simulink model "OrientationAnimationModel"  (R2023b)
settings: Solver=ode3  StartTime=0.0  StopTime=500  FixedStep=.010  RelTol=1e-3
model workspace (MAT data in the model file):
  B = Simulink.Parameter
  B.Value = Simulink.data.Expression
  B.Value.ExpressionString = "3.42*(1e-6)/((2*pi/60)*1e3)"
  B.DataType = 'auto'
  B.Complexity = 'real'
  B.Dimensions = -1
  J = Simulink.Parameter
  J.Value = Simulink.data.Expression
  J.Value.ExpressionString = "0.5*0.05*(0.05)^2"
  J.DataType = 'auto'
  J.Complexity = 'real'
  J.Dimensions = -1
  Kt = Simulink.Parameter
  Kt.Value = Simulink.data.Expression
  Kt.Value.ExpressionString = "3.56*1e-3"
  Kt.DataType = 'auto'
  Kt.Complexity = 'real'
  Kt.Dimensions = -1
  L = Simulink.Parameter
  L.Value = Simulink.data.Expression
  L.Value.ExpressionString = "570*1e-6"
  L.DataType = 'auto'
  L.Complexity = 'real'
  L.Dimensions = -1
  M1_Gain = Simulink.Parameter
  M1_Gain.Value = 8.4
  M1_Gain.DataType = 'auto'
  M1_Gain.Complexity = 'real'
  M1_Gain.Dimensions = [1 1]
  M1_I_max = Simulink.Parameter
  M1_I_max.Value = 0.075
  M1_I_max.DataType = 'auto'
  M1_I_max.Complexity = 'real'
  M1_I_max.Dimensions = [1 1]
  M1_V = Simulink.Parameter
  M1_V.Value = 5
  M1_V.DataType = 'auto'
  M1_V.Complexity = 'real'
  M1_V.Dimensions = [1 1]
  M2_Gain = Simulink.Parameter
  M2_Gain.Value = 8.4
  M2_Gain.DataType = 'auto'
  M2_Gain.Complexity = 'real'
  M2_Gain.Dimensions = [1 1]
  M2_I_max = Simulink.Parameter
  M2_I_max.Value = 0.075
  M2_I_max.DataType = 'auto'
  M2_I_max.Complexity = 'real'
  M2_I_max.Dimensions = [1 1]
  M2_V = Simulink.Parameter
  M2_V.Value = 5
  M2_V.DataType = 'auto'
  M2_V.Complexity = 'real'
  M2_V.Dimensions = [1 1]
  R = Simulink.Parameter
  R.Value = Simulink.data.Expression
  R.Value.ExpressionString = "22"
  R.DataType = 'auto'
  R.Complexity = 'real'
  R.Dimensions = -1
  orbit_altitude = 450000
  r_earth = 6378100
  vel_init = 7640
undefined symbols (not defined in the file or in its folder): m1, m2, m3, V1, V2, V3
libraries: aerolibutil x5, dspinverses x4, sharedtransform x4, simulink x3, vrlib x1, dspmtrx3 x1, matrix_library x1, spsSampleandHoldLib x1
settings Model: SnapshotInterval=1  Creator=Ian Lee  LastModifiedBy=andrea
settings DebuggingCC: UnconnectedInputMsg=warning  UnconnectedOutputMsg=warning  UnconnectedLineMsg=warning
settings ModelReferenceCC: EnableRefExpFcnMdlSchedulingChecks=on  ModelReferenceMinAlgLoopOccurrences=on
settings RTWCC: DLArmComputeVersion=19.05

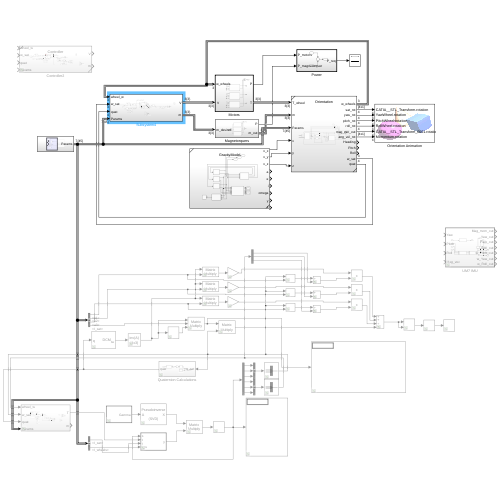
[thumbnail: Simulink's stored preview of the top-level diagram]
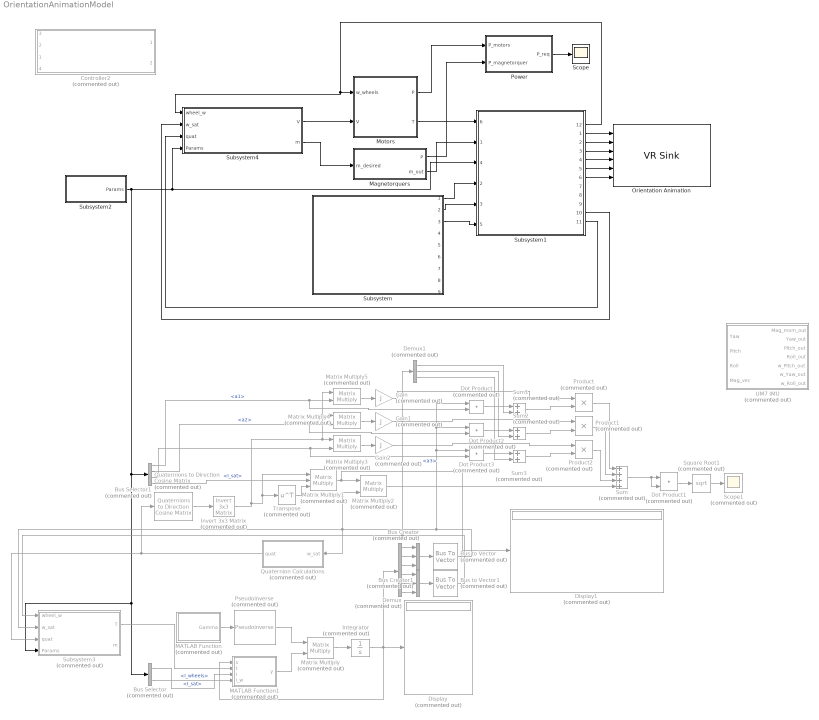
== system OrientationAnimationModel ==
  Bus Creator : BusCreator  Commented=on  Inputs=3
  Bus Creator1 : BusCreator  Commented=on  Inputs=3
  Bus Selector : BusSelector  Commented=on  OutputSignals=I_sat,I_wheels
  Bus Selector1 : BusSelector  Commented=on  OutputSignals=a1,a2,a3,I_sat
  Bus to Vector : BusToVector  Commented=on
  Bus to Vector1 : BusToVector  Commented=on
  Controller2 : Subsystem  Commented=on  ReferencedSubsystem=Controller
      settings: PortSchema="{\"entries\":[{\"content\":{\"sides\":[{\"content\":{\"connectorIds\":[\"In3\",\"In2\",\"In1\",\"In4\"]},\"type\":\"ConnectorPlacement.EquallySpacedRectSide\",\"uuid\":\"79f889b4-4a86-42cb-9f90-6ea385053cf3\"},{\"content\":{\"connectorIds\":[\"Out1\",\"Out2\"],\"side\":\"RIGHT\"},\"type\":\"ConnectorPlacement.EquallySpacedRectSide\",\"uuid\":\"c6c22cdf-cbb6-43f0-a5d1-c6e13417ad06\"},{\"content\":{\"side\":\"TOP\"},\"type\":\"ConnectorPlacement.EquallySpacedRectSide\",\"uuid\":\"fe3f8c93-2b15-4833-a3bc-63f563fd4268\"}]},\"type\":\"ConnectorPlacement.EquallySpacedConnector\",\"uuid\":\"198af49c-de07-4ebb-ae2e-d5790619fe38\"}],\"packageUris\":[\"http://schema.mathworks.com/mf0/Connector/R2020b\"],\"version\":\"1.0\"}"
  Demux : Demux  Commented=on  Outputs=6
  Demux1 : Demux  Commented=on  Outputs=3
  Display : Display  Commented=on
  Display1 : Display  Commented=on
  Dot Product{,1..3} (4 alike) : DotProduct  Commented=on  OutDataTypeStr=Inherit: Inherit via internal rule
  Gain : Gain  Commented=on  Gain=J
  Gain1 : Gain  Commented=on  Gain=J
  Gain2 : Gain  Commented=on  Gain=J
  Integrator : Integrator  Commented=on  InitialCondition=[0;0;0;0;0;0]
  Invert 3x3 Matrix : aerolibutil/Invert  3x3 Matrix  Commented=on
  MATLAB Function : MATLAB Function  Commented=on  TreatAsAtomicUnit=on
  MATLAB Function1 : MATLAB Function  Commented=on  TreatAsAtomicUnit=on
  Magnetorquers : Subsystem
  Matrix Multiply{,2..5} (5 alike) : Product  Commented=on  Multiplication=Matrix(*)
  Matrix Multiply1 : Product  Commented=on  Inputs=3  Multiplication=Matrix(*)
  Motors : Subsystem  TreatAsAtomicUnit=on
  Orientation Animation : vrlib/VR Sink  InstantiateOnLoad=on  SampleTime=.02  ViewEnable=on  RemoteChange=off  RemoteView=off  FieldsWritten=CATIA__STL_Transform.rotation.4.1.1.double#YawWheel.rotation.4.1.1.double#PitchWheel.rotation.4.1.1.double#RollWheel.rotation.4.1.1.double#CATIA__STL_Transform_0001.rotation.4.1.1.double#Momentum.rotation.4.1.1.double  WorldFileName=SatVR.x3d  AutoView=off  VideoDimensions=[]  AllowVariableSize=off
  Power : Subsystem  TreatAsAtomicUnit=on
  Product : Product  Commented=on
  Product1 : Product  Commented=on
  Product2 : Product  Commented=on
  Pseudoinverse : dspinverses/Pseudoinverse  Commented=on  wanterr=off  SimulateUsing=Interpreted execution
  Quaternion Calculations : Subsystem  Commented=on
  Quaternions to Direction Cosine Matrix : sharedtransform/Quaternions to  Direction Cosine Matrix  Commented=on  aMode=aMode
      settings: LibrarySourceBlock=|
      | aerolibtransform2/Quaternions to
      | Direction Cosine Matrix
  Scope : Scope
  Scope1 : Scope  Commented=on
  Square Root1 : Sqrt  Commented=on
  Subsystem : Subsystem  ReferencedSubsystem=GravityModel
  Subsystem1 : Subsystem  ReferencedSubsystem=Orientation
      settings: PortSchema="{\"entries\":[{\"content\":{\"sides\":[{\"content\":{\"connectorIds\":[\"In6\",\"In1\",\"In4\",\"In2\",\"In3\",\"In5\"]},\"type\":\"ConnectorPlacement.EquallySpacedRectSide\",\"uuid\":\"8242cc14-2b60-48ca-86c2-9381cf9d168d\"},{\"content\":{\"connectorIds\":[\"Out12\",\"Out1\",\"Out2\",\"Out3\",\"Out4\",\"Out5\",\"Out6\",\"Out7\",\"Out8\",\"Out9\",\"Out10\",\"Out11\"],\"side\":\"RIGHT\"},\"type\":\"ConnectorPlacement.EquallySpacedRectSide\",\"uuid\":\"8dac9f9e-c84b-46a7-8096-472338eb4c0b\"},{\"content\":{\"side\":\"TOP\"},\"type\":\"ConnectorPlacement.EquallySpacedRectSide\",\"uuid\":\"ad35a777-644b-4799-a01f-486ba56fdd07\"}]},\"type\":\"ConnectorPlacement.EquallySpacedConnector\",\"uuid\":\"a47ae8ba-a922-42d0-80de-66716a9fad33\"}],\"packageUris\":[\"http://schema.mathworks.com/mf0/Connector/R2020b\"],\"version\":\"1.0\"}"
  Subsystem2 : Subsystem
  Subsystem3 : Subsystem  Commented=on
  Subsystem4 : Subsystem
  Sum : Sum  Commented=on  Inputs=++++
  Sum1 : Sum  Commented=on
  Sum2 : Sum  Commented=on
  Sum3 : Sum  Commented=on
  Transpose : Math  Commented=on  Operator=transpose
  UM7 IMU : Subsystem  Commented=on  TreatAsAtomicUnit=on
  wires:
  Subsystem/1 -> Subsystem1/2
  Subsystem/2 -> Subsystem1/3
  Subsystem/3 -> Subsystem1/5
  Power/1(P_req) -> Scope/1
  Magnetorquers/1(P) -> Power/2(P_magnetorquer)
  Subsystem1/1 -> Orientation Animation/1
  Subsystem1/2 -> Orientation Animation/2
  Subsystem1/3 -> Orientation Animation/3
  Subsystem1/4 -> Orientation Animation/4
  Subsystem1/5 -> Orientation Animation/5
  Subsystem1/6 -> Orientation Animation/6
  Subsystem1/11 -> Subsystem4/3(quat)
  Subsystem1/10 -> Subsystem4/2(w_sat)
  Subsystem4/1(V) -> Motors/2(" V")
  Subsystem4/2(m) -> Magnetorquers/1(m_desired)
  Magnetorquers/2(m_out) -> Subsystem1/1
  Motors/1(P) -> Power/1(P_motors)
  Motors/2(T) -> Subsystem1/6
  Subsystem1/12 -> Subsystem4/1(wheel_w), Motors/1(w_wheels)
  Subsystem2/1(Params) -> Subsystem4/4(Params), Subsystem1/4, Bus Selector1/1, Subsystem3/4(Params), Bus Selector/1
  MATLAB Function/1(Gamma) -> Pseudoinverse/1
  Pseudoinverse/1 -> Matrix Multiply/1
  MATLAB Function1/1(y) -> Matrix Multiply/2
  Matrix Multiply/1 -> Integrator/1
  Integrator/1 -> Demux/1, MATLAB Function1/1(s), Display/1
  Bus Selector/1 -> MATLAB Function1/3(I)  "<I_sat>"
  Bus Selector/2 -> MATLAB Function1/4(I_w)  "<I_wheels>"
  Demux/1 -> Bus Creator/1
  Demux/2 -> Bus Creator/2
  Demux/3 -> Bus Creator/3
  Demux/4 -> Bus Creator1/1
  Demux/5 -> Bus Creator1/2
  Demux/6 -> Bus Creator1/3
  Bus Creator/1 -> Bus to Vector/1
  Bus Creator1/1 -> Bus to Vector1/1
  Bus to Vector/1 -> Dot Product3/1, Dot Product2/1, Dot Product/1, Matrix Multiply2/2, Quaternion Calculations/1(w_sat), Subsystem3/2(w_sat)
  Bus to Vector1/1 -> Demux1/1, Subsystem3/1(wheel_w)
  Quaternion Calculations/1(quat) -> Quaternions to Direction Cosine Matrix/1, Subsystem3/3(quat)
  Subsystem3/1(T) -> MATLAB Function1/2(t)
  Transpose/1 -> Matrix Multiply1/3
  Matrix Multiply1/1 -> Display1/1, Matrix Multiply2/1
  Bus Selector1/4 -> Matrix Multiply1/2  "<I_sat>"
  Bus Selector1/3 -> Dot Product3/2, Matrix Multiply3/2  "<a3>"
  Bus Selector1/2 -> Dot Product2/2, Matrix Multiply4/2  "<a2>"
  Bus Selector1/1 -> Dot Product/2, Matrix Multiply5/2  "<a1>"
  Matrix Multiply3/1 -> Gain2/1
  Matrix Multiply5/1 -> Gain/1
  Matrix Multiply4/1 -> Gain1/1
  Gain/1 -> Product/1
  Gain1/1 -> Product1/1
  Gain2/1 -> Product2/1
  Matrix Multiply2/1 -> Sum/4
  Product2/1 -> Sum/3
  Product1/1 -> Sum/2
  Product/1 -> Sum/1
  Sum/1 -> Dot Product1/2, Dot Product1/1
  Dot Product1/1 -> Square Root1/1
  Square Root1/1 -> Scope1/1
  Dot Product/1 -> Sum1/1
  Dot Product2/1 -> Sum2/1
  Dot Product3/1 -> Sum3/1
  Demux1/1 -> Sum1/2
  Demux1/2 -> Sum2/2
  Demux1/3 -> Sum3/2
  Sum1/1 -> Product/2
  Sum2/1 -> Product1/2
  Sum3/1 -> Product2/2
  Quaternions to Direction Cosine Matrix/1 -> Invert 3x3 Matrix/1
  Invert 3x3 Matrix/1 -> Matrix Multiply5/1, Matrix Multiply4/1, Matrix Multiply3/1, Transpose/1, Matrix Multiply1/1

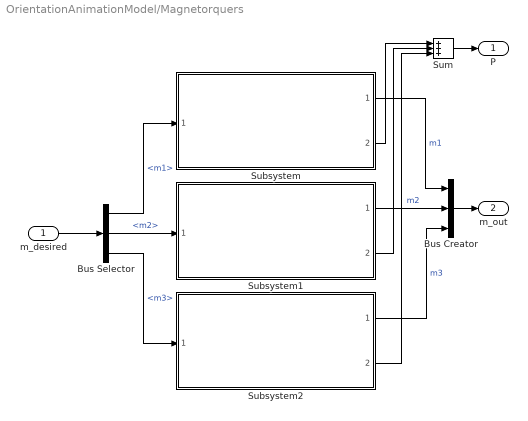
== system OrientationAnimationModel/Magnetorquers ==
  m_desired : Inport
  Bus Creator : BusCreator  Inputs=m1,m2,m3
  Bus Selector : BusSelector  OutputSignals=m1,m2,m3
  Subsystem : Subsystem  ReferencedSubsystem=Magnetorquer  M_s=1.6E+6  a=1100  n=1000  k=400  R=4.0416  c=0.2  L=0.1  alpha=0.0016  A_=0.00020106192  mu_0=1.25663706212E-6
  Subsystem1 : Subsystem  ReferencedSubsystem=Magnetorquer  M_s=1.6E+6  a=1100  n=1000  k=400  R=4.0416  c=0.2  L=0.1  alpha=0.0016  A_=0.00020106192  mu_0=1.25663706212E-6
  Subsystem2 : Subsystem  ReferencedSubsystem=Magnetorquer  M_s=1.6E+6  a=1100  n=1000  k=400  R=4.0416  c=0.2  L=0.1  alpha=0.0016  A_=0.00020106192  mu_0=1.25663706212E-6
  Sum : Sum  Inputs=+++
  P : Outport
  m_out : Outport  Port=2
  wires:
  Bus Selector/2 -> Subsystem1/1  "<m2>"
  Bus Selector/3 -> Subsystem2/1  "<m3>"
  Subsystem/1 -> Bus Creator/1  "m1"
  Subsystem1/1 -> Bus Creator/2  "m2"
  Subsystem2/1 -> Bus Creator/3  "m3"
  Subsystem/2 -> Sum/1
  Subsystem1/2 -> Sum/2
  Subsystem2/2 -> Sum/3
  Sum/1 -> P/1
  m_desired/1 -> Bus Selector/1
  Bus Selector/1 -> Subsystem/1  "<m1>"
  Bus Creator/1 -> m_out/1

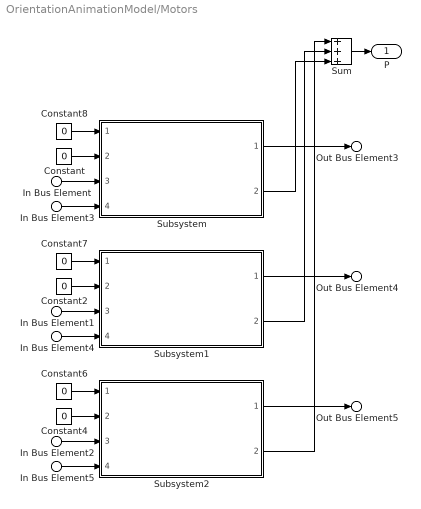
== system OrientationAnimationModel/Motors ==
  In Bus Element3 : Inport  PortName=w_wheels  Element=w_wheel1
  In Bus Element4 : Inport  PortName=w_wheels  Element=w_wheel2
  In Bus Element5 : Inport  PortName=w_wheels  Element=w_wheel3
  In Bus Element : Inport  Port=2  PortName=V  Element=V1
  In Bus Element1 : Inport  Port=2  PortName=V  Element=V2
  In Bus Element2 : Inport  Port=2  PortName=V  Element=V3
  Constant{,2,4,6..8} (6 alike) : Constant  Value=0
  Subsystem : Subsystem  ReferencedSubsystem=DCMotorTorqueModel  T_max=0.000953  w_max=1570.79632679  V_max=6  Kt=0.00356
  Subsystem1 : Subsystem  ReferencedSubsystem=DCMotorTorqueModel  T_max=0.000953  w_max=1570.79632679  V_max=6  Kt=0.00356
  Subsystem2 : Subsystem  ReferencedSubsystem=DCMotorTorqueModel  T_max=0.000953  w_max=1570.79632679  V_max=6  Kt=0.00356
  Sum : Sum  Inputs=+++
  P : Outport
  Out Bus Element3 : Outport  Port=2  PortName=T  Element=T1
  Out Bus Element4 : Outport  Port=2  PortName=T  Element=T2
  Out Bus Element5 : Outport  Port=2  PortName=T  Element=T3
  wires:
  Constant/1 -> Subsystem/2
  Constant2/1 -> Subsystem1/2
  Constant4/1 -> Subsystem2/2
  Constant6/1 -> Subsystem2/1
  Constant7/1 -> Subsystem1/1
  Constant8/1 -> Subsystem/1
  In Bus Element3/1 -> Subsystem/4
  In Bus Element4/1 -> Subsystem1/4
  In Bus Element5/1 -> Subsystem2/4
  Sum/1 -> P/1
  In Bus Element/1 -> Subsystem/3
  In Bus Element1/1 -> Subsystem1/3
  In Bus Element2/1 -> Subsystem2/3
  Subsystem/2 -> Sum/3
  Subsystem1/2 -> Sum/2
  Subsystem2/2 -> Sum/1
  Subsystem/1 -> Out Bus Element3/1
  Subsystem1/1 -> Out Bus Element4/1
  Subsystem2/1 -> Out Bus Element5/1

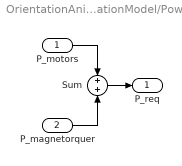
== system OrientationAnimationModel/Power ==
  P_motors : Inport
  P_magnetorquer : Inport  Port=2
  Sum : Sum
  P_req : Outport
  wires:
  Sum/1 -> P_req/1
  P_magnetorquer/1 -> Sum/2
  P_motors/1 -> Sum/1

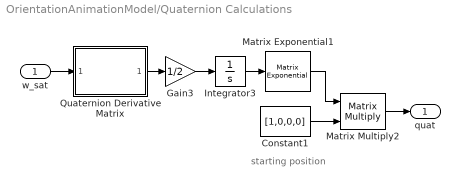
== system OrientationAnimationModel/Quaternion Calculations ==
  note: starting position
  w_sat : Inport
  Constant1 : Constant  Value=[1,0,0,0]
  Gain3 : Gain  Gain=1/2
  Integrator3 : Integrator  InitialCondition=[[0,0,0,0];[0,0,0,0];[0,0,0,0];[0,0,0,0]]
  Matrix Exponential1 : dspmtrx3/Matrix Exponential
  Matrix Multiply2 : Product  Multiplication=Matrix(*)
  Quaternion Derivative Matrix : MATLAB Function  TreatAsAtomicUnit=on
  quat : Outport
  wires:
  Quaternion Derivative Matrix/1(Omega) -> Gain3/1
  Gain3/1 -> Integrator3/1
  Matrix Exponential1/1 -> Matrix Multiply2/1
  Constant1/1 -> Matrix Multiply2/2
  Integrator3/1 -> Matrix Exponential1/1
  Matrix Multiply2/1 -> quat/1
  w_sat/1 -> Quaternion Derivative Matrix/1(omega)

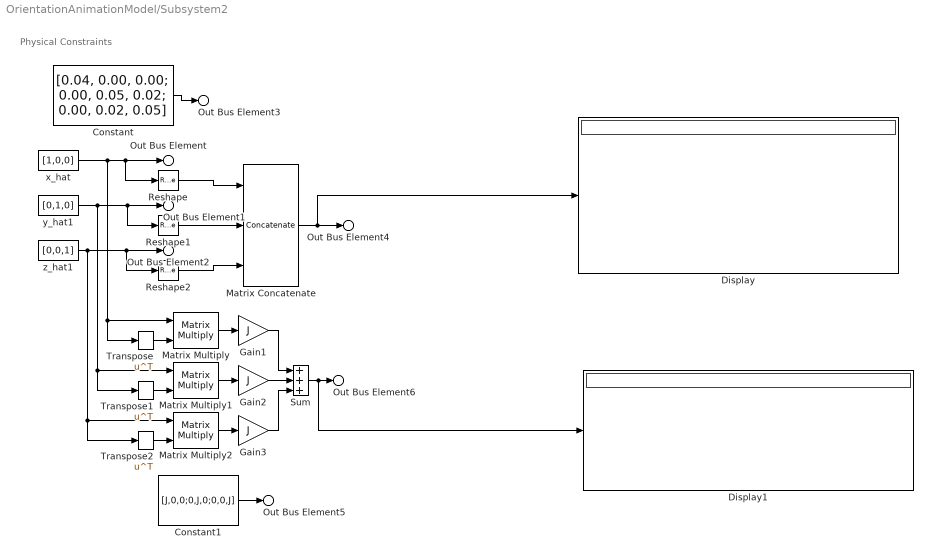
== system OrientationAnimationModel/Subsystem2 ==
  note: Physical Constraints
  Constant : Constant  Value=|
      | [0.04, 0.00, 0.00;
      | 0.00, 0.05, 0.02;
      | 0.00, 0.02, 0.05]
  Constant1 : Constant  Value=[J,0,0;0,J,0;0,0,J]
  Display : Display
  Display1 : Display
  Gain1 : Gain  Gain=J
  Gain2 : Gain  Gain=J
  Gain3 : Gain  Gain=J
  Matrix Concatenate : Concatenate  NumInputs=3  Mode=Multidimensional array  ConcatenateDimension=2
  Matrix Multiply : Product  Multiplication=Matrix(*)
  Matrix Multiply1 : Product  Multiplication=Matrix(*)
  Matrix Multiply2 : Product  Multiplication=Matrix(*)
  Reshape : Reshape  OutputDimensionality=Customize  OutputDimensions=[3,1]
  Reshape1 : Reshape  OutputDimensionality=Customize  OutputDimensions=[3,1]
  Reshape2 : Reshape  OutputDimensionality=Customize  OutputDimensions=[3,1]
  Sum : Sum  Inputs=+++
  Transpose : Math  Operator=transpose
  Transpose1 : Math  Operator=transpose
  Transpose2 : Math  Operator=transpose
  x_hat : Constant  Value=[1,0,0]
  y_hat1 : Constant  Value=[0,1,0]
  z_hat1 : Constant  Value=[0,0,1]
  Out Bus Element : Outport  PortName=Params  Element=a1
  Out Bus Element1 : Outport  PortName=Params  Element=a2
  Out Bus Element2 : Outport  PortName=Params  Element=a3
  Out Bus Element3 : Outport  PortName=Params  Element=I_sat
  Out Bus Element4 : Outport  PortName=Params  Element=A
  Out Bus Element5 : Outport  PortName=Params  Element=I_wheels
  Out Bus Element6 : Outport  PortName=Params  Element=wheel_mat
  wires:
  z_hat1/1 -> Transpose2/1, Matrix Multiply2/1, Reshape2/1, Out Bus Element2/1
  x_hat/1 -> Transpose/1, Matrix Multiply/1, Reshape/1, Out Bus Element/1
  Constant/1 -> Out Bus Element3/1
  y_hat1/1 -> Transpose1/1, Matrix Multiply1/1, Reshape1/1, Out Bus Element1/1
  Reshape/1 -> Matrix Concatenate/1
  Reshape1/1 -> Matrix Concatenate/2
  Reshape2/1 -> Matrix Concatenate/3
  Matrix Concatenate/1 -> Display/1, Out Bus Element4/1
  Transpose/1 -> Matrix Multiply/2
  Transpose1/1 -> Matrix Multiply1/2
  Transpose2/1 -> Matrix Multiply2/2
  Matrix Multiply/1 -> Gain1/1
  Matrix Multiply1/1 -> Gain2/1
  Gain2/1 -> Sum/2
  Gain1/1 -> Sum/1
  Gain3/1 -> Sum/3
  Sum/1 -> Out Bus Element6/1, Display1/1
  Matrix Multiply2/1 -> Gain3/1
  Constant1/1 -> Out Bus Element5/1

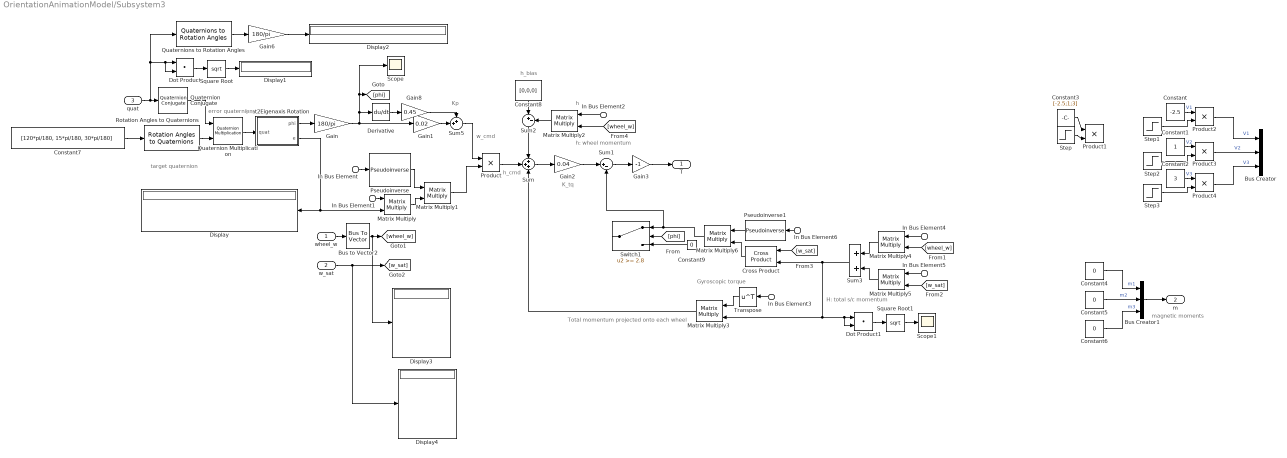
== system OrientationAnimationModel/Subsystem3 ==
  note: H: total s/c momentum
  note: h: wheel momentum
  note: w_cmd
  note: Kp
  note: magnetic moments
  note: h_bias
  note: target quaternion
  note: h_cmd
  note: K_tq
  note: error quaternion
  note: h
  note: Gyroscopic torque
  note: Total momentum projected onto each wheel
  wheel_w : Inport
  w_sat : Inport  Port=2  PortDimensions=3
  quat : Inport  Port=3  PortDimensions=4
  In Bus Element : Inport  Port=4  PortName=Params  Element=A
  In Bus Element3 : Inport  Port=4  PortName=Params  Element=A
  In Bus Element6 : Inport  Port=4  PortName=Params  Element=A
  In Bus Element1 : Inport  Port=4  PortName=Params  Element=I_sat
  In Bus Element5 : Inport  Port=4  PortName=Params  Element=I_sat
  In Bus Element2 : Inport  Port=4  PortName=Params  Element=I_wheels
  In Bus Element4 : Inport  Port=4  PortName=Params  Element=I_wheels
  Bus Creator : BusCreator  Inputs=3
  Bus Creator1 : BusCreator  Inputs=m1,m2,m3
  Bus to Vector2 : BusToVector
  Constant : Constant  Value=-2.5
  Constant1 : Constant
  Constant2 : Constant  Value=3
  Constant3 : Constant  Value=[-2.5;1;3]
  Constant{4..6,9} (4 alike) : Constant  Value=0
  Constant7 : Constant  Value=[120*pi/180, 15*pi/180, 30*pi/180]  VectorParams1D=off
  Constant8 : Constant  Value=[0,0,0]
  Cross Product : matrix_library/Cross Product
  Derivative : Derivative
  Display{,1..4} (5 alike) : Display
  Dot Product : DotProduct  OutDataTypeStr=Inherit: Inherit via internal rule
  Dot Product1 : DotProduct  OutDataTypeStr=Inherit: Inherit via internal rule
  Gain : Gain  Gain=180/pi
  Gain1 : Gain  Gain=0.02
  Gain2 : Gain  Gain=0.04
  Gain3 : Gain  Gain=-1
  Gain6 : Gain  Gain=180/pi
  Gain8 : Gain  Gain=0.45
  Matrix Multiply{,1..6} (7 alike) : Product  Multiplication=Matrix(*)
  Product{,1..4} (5 alike) : Product
  Pseudoinverse : dspinverses/Pseudoinverse  wanterr=off  SimulateUsing=Interpreted execution
  Pseudoinverse1 : dspinverses/Pseudoinverse  wanterr=off  SimulateUsing=Interpreted execution
  Quat2Eigenaxis Rotation : MATLAB Function  TreatAsAtomicUnit=on
  Quaternion Conjugate : aerolibutil/Quaternion Conjugate
  Quaternion Multiplication : aerolibutil/Quaternion Multiplication
  Quaternions to Rotation Angles : sharedtransform/Quaternions to Rotation Angles  rotationOrder=ZYX  aMode=aMode
  Rotation Angles to Quaternions : sharedtransform/Rotation Angles to Quaternions  rotationOrder=ZYX  aMode=aMode
  Scope : Scope
  Scope1 : Scope
  Square Root : Sqrt
  Square Root1 : Sqrt
  Step : Step  Before=1  After=-1  SampleTime=0
  Step1 : Step  Time=2  Before=1  After=-1  SampleTime=0
  Step2 : Step  Time=2  Before=1  After=-1  SampleTime=0
  Step3 : Step  Time=2  Before=1  After=-1  SampleTime=0
  Sum : Sum  Inputs=+++
  Sum1 : Sum  Inputs=|+-
  Sum2 : Sum  Inputs=|+-
  Sum3 : Sum
  Sum5 : Sum  Inputs=++|
  Switch1 : Switch  Threshold=2.8  SaturateOnIntegerOverflow=off  InputSameDT=off
  Transpose : Math  Operator=transpose
  T : Outport
  m : Outport  Port=2
  wires:
  Quaternion Conjugate/1 -> Quaternion Multiplication/1
  Sum1/1 -> Gain3/1
  Sum3/1 -> Dot Product1/2, Dot Product1/1, Matrix Multiply3/2, Cross Product/2
  [phi] -> Switch1/2
  Derivative/1 -> Gain8/1
  Constant/1 -> Product2/1  "V1"
  [w_sat] -> Matrix Multiply5/2
  Dot Product1/1 -> Square Root1/1
  w_sat/1 -> Display4/1, [w_sat]
  wheel_w/1 -> Bus to Vector2/1
  Matrix Multiply1/1 -> Product/2
  [wheel_w] -> Matrix Multiply4/2
  In Bus Element4/1 -> Matrix Multiply4/1
  Matrix Multiply4/1 -> Sum3/1
  Transpose/1 -> Matrix Multiply3/1
  Sum2/1 -> Sum/1
  Quat2Eigenaxis Rotation/2(e) -> Matrix Multiply/2, Display/1
  [wheel_w] -> Matrix Multiply2/2
  In Bus Element1/1 -> Matrix Multiply/1
  In Bus Element/1 -> Pseudoinverse/1
  Constant4/1 -> Bus Creator1/1  "m1"
  Constant5/1 -> Bus Creator1/2  "m2"
  Constant6/1 -> Bus Creator1/3  "m3"
  Quat2Eigenaxis Rotation/1(phi) -> Gain/1
  Rotation Angles to Quaternions/1 -> Quaternion Multiplication/2
  Gain/1 -> Gain1/1, Scope/1, [phi], Derivative/1
  Constant8/1 -> Sum2/1
  Constant2/1 -> Product4/1  "V3"
  Matrix Multiply6/1 -> Sum1/2, Switch1/1
  Step2/1 -> Product3/2
  Step/1 -> Product1/2
  Bus to Vector2/1 -> Display3/1, [wheel_w]
  Step3/1 -> Product4/2
  Product4/1 -> Bus Creator/3  "V3"
  Product3/1 -> Bus Creator/2  "V2"
  quat/1 -> Dot Product/2, Dot Product/1, Quaternions to Rotation Angles/1, Quaternion Conjugate/1
  Product2/1 -> Bus Creator/1  "V1"
  Constant3/1 -> Product1/1
  Cross Product/1 -> Matrix Multiply6/2
  Step1/1 -> Product2/2
  Constant1/1 -> Product3/1  "V2"
  Pseudoinverse/1 -> Matrix Multiply1/1
  Quaternion Multiplication/1 -> Quat2Eigenaxis Rotation/1(quat)
  [w_sat] -> Cross Product/1
  Constant9/1 -> Switch1/3
  Square Root1/1 -> Scope1/1
  Constant7/1 -> Rotation Angles to Quaternions/1
  In Bus Element5/1 -> Matrix Multiply5/1
  Bus Creator1/1 -> m/1
  In Bus Element6/1 -> Pseudoinverse1/1
  Sum/1 -> Gain2/1
  Gain2/1 -> Sum1/1
  Pseudoinverse1/1 -> Matrix Multiply6/1
  Gain6/1 -> Display2/1
  In Bus Element2/1 -> Matrix Multiply2/1
  Product/1 -> Sum/2
  Matrix Multiply2/1 -> Sum2/2
  Quaternions to Rotation Angles/1 -> Gain6/1
  In Bus Element3/1 -> Transpose/1
  Gain1/1 -> Sum5/2
  Gain8/1 -> Sum5/1
  Dot Product/1 -> Square Root/1
  Matrix Multiply/1 -> Matrix Multiply1/2
  Matrix Multiply3/1 -> Sum/3
  Square Root/1 -> Display1/1
  Matrix Multiply5/1 -> Sum3/2
  Sum5/1 -> Product/1
  Gain3/1 -> T/1

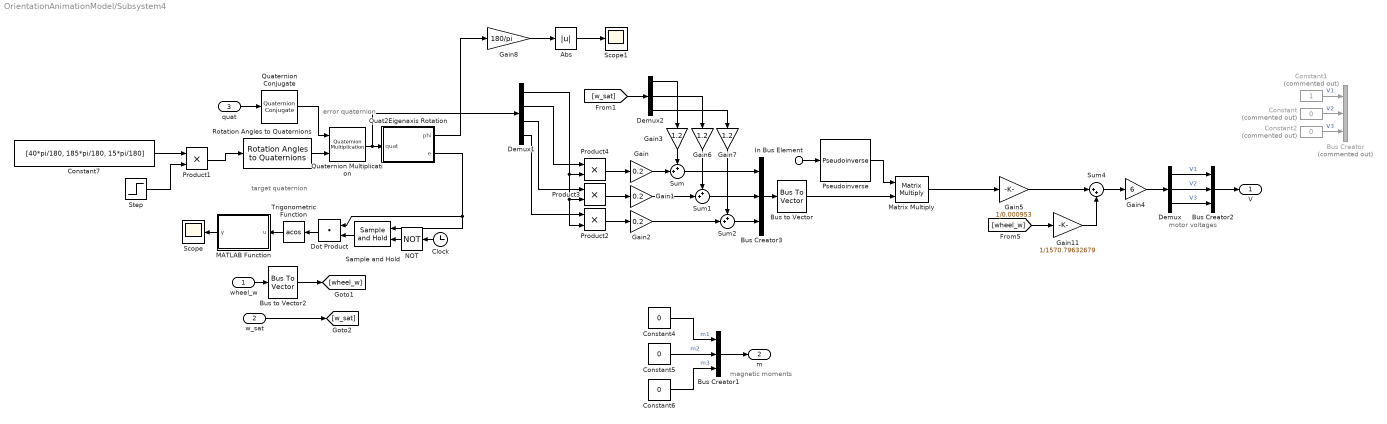
== system OrientationAnimationModel/Subsystem4 ==
  note: motor voltages
  note: target quaternion
  note: error quaternion
  note: magnetic moments
  wheel_w : Inport
  w_sat : Inport  Port=2  PortDimensions=3
  quat : Inport  Port=3  PortDimensions=4
  In Bus Element : Inport  Port=4  PortName=Params  Element=A
  Abs : Abs  SaturateOnIntegerOverflow=off
  Bus Creator : BusCreator  Commented=on  Inputs=3
  Bus Creator1 : BusCreator  Inputs=m1,m2,m3
  Bus Creator2 : BusCreator  Inputs=V1,V2,V3
  Bus Creator3 : BusCreator  Inputs=3
  Bus to Vector : BusToVector
  Bus to Vector2 : BusToVector
  Clock : Clock
  Constant : Constant  Commented=on  Value=0
  Constant1 : Constant  Commented=on
  Constant2 : Constant  Commented=on  Value=0
  Constant4 : Constant  Value=0
  Constant5 : Constant  Value=0
  Constant6 : Constant  Value=0
  Constant7 : Constant  Value=[40*pi/180, 185*pi/180, 15*pi/180]  VectorParams1D=off
  Demux : Demux  Outputs=3
  Demux1 : Demux
  Demux2 : Demux  Outputs=3
  Dot Product : DotProduct  OutDataTypeStr=Inherit: Inherit via internal rule
  Gain : Gain  Gain=0.2
  Gain1 : Gain  Gain=0.2
  Gain11 : Gain  Gain=1/1570.79632679
  Gain2 : Gain  Gain=0.2
  Gain3 : Gain  Gain=1.2
  Gain4 : Gain  Gain=6  OutMin=-6  OutMax=6
  Gain5 : Gain  Gain=1/0.000953
  Gain6 : Gain  Gain=1.2
  Gain7 : Gain  Gain=1.2
  Gain8 : Gain  Gain=180/pi
  MATLAB Function : MATLAB Function  TreatAsAtomicUnit=on
  Matrix Multiply : Product  Multiplication=Matrix(*)
  NOT : Logic  Operator=NOT  IconShape=distinctive  AllPortsSameDT=off  OutDataTypeStr=boolean
  Product{1..4} (4 alike) : Product
  Pseudoinverse : dspinverses/Pseudoinverse  wanterr=off  SimulateUsing=Interpreted execution
  Quat2Eigenaxis Rotation : MATLAB Function  TreatAsAtomicUnit=on
  Quaternion Conjugate : aerolibutil/Quaternion Conjugate
  Quaternion Multiplication : aerolibutil/Quaternion Multiplication
  Rotation Angles to Quaternions : sharedtransform/Rotation Angles to Quaternions  rotationOrder=ZYX  aMode=aMode
  Sample and Hold : spsSampleandHoldLib/Sample and Hold  ic=0  Ts=0
      settings: LibrarySourceBlock=|
      | sps_lib/Control/Sample and
      | Hold
  Scope : Scope
  Scope1 : Scope
  Step : Step  Time=10  Before=1  SampleTime=0
  Sum : Sum  Inputs=++|
  Sum1 : Sum  Inputs=++|
  Sum2 : Sum  Inputs=++|
  Sum4 : Sum  Inputs=|++
  Trigonometric Function : Trigonometry  Operator=acos
  V : Outport
  m : Outport  Port=2
  wires:
  Constant1/1 -> Bus Creator/1  "V1"
  Bus to Vector2/1 -> [wheel_w]
  Quaternion Multiplication/1 -> Demux1/1, Quat2Eigenaxis Rotation/1(quat)
  Clock/1 -> NOT/1
  Demux/3 -> Bus Creator2/3  "V3"
  Rotation Angles to Quaternions/1 -> Quaternion Multiplication/2
  Sum4/1 -> Gain4/1
  [wheel_w] -> Gain11/1
  Demux/1 -> Bus Creator2/1  "V1"
  Quat2Eigenaxis Rotation/1(phi) -> Gain8/1
  Dot Product/1 -> Trigonometric Function/1
  w_sat/1 -> [w_sat]
  wheel_w/1 -> Bus to Vector2/1
  Gain11/1 -> Sum4/2
  Constant2/1 -> Bus Creator/3  "V3"
  Constant5/1 -> Bus Creator1/2  "m2"
  Demux/2 -> Bus Creator2/2  "V2"
  Trigonometric Function/1 -> MATLAB Function/1(u)
  Constant/1 -> Bus Creator/2  "V2"
  Bus Creator2/1 -> V/1
  quat/1 -> Quaternion Conjugate/1
  Constant6/1 -> Bus Creator1/3  "m3"
  Constant4/1 -> Bus Creator1/1  "m1"
  Gain4/1 -> Demux/1
  Quaternion Conjugate/1 -> Quaternion Multiplication/1
  Gain5/1 -> Sum4/1
  NOT/1 -> Sample and Hold/2
  Quat2Eigenaxis Rotation/2(e) -> Dot Product/1, Sample and Hold/1
  MATLAB Function/1(y) -> Scope/1
  Product1/1 -> Rotation Angles to Quaternions/1
  Sample and Hold/1 -> Dot Product/2
  Constant7/1 -> Product1/1
  Bus Creator1/1 -> m/1
  Step/1 -> Product1/2
  Product4/1 -> Gain/1
  Product3/1 -> Gain1/1
  Product2/1 -> Gain2/1
  Gain/1 -> Sum/2
  Gain1/1 -> Sum1/2
  Gain2/1 -> Sum2/2
  [w_sat] -> Demux2/1
  Demux2/1 -> Gain3/1
  Demux2/2 -> Gain6/1
  Demux2/3 -> Gain7/1
  Sum/1 -> Bus Creator3/1
  Sum1/1 -> Bus Creator3/2
  Sum2/1 -> Bus Creator3/3
  Bus Creator3/1 -> Bus to Vector/1
  In Bus Element/1 -> Pseudoinverse/1
  Bus to Vector/1 -> Matrix Multiply/2
  Pseudoinverse/1 -> Matrix Multiply/1
  Gain8/1 -> Abs/1
  Matrix Multiply/1 -> Gain5/1
  Demux1/2 -> Product4/1
  Demux1/3 -> Product3/1
  Demux1/4 -> Product2/1
  Demux1/1 -> Product2/2, Product3/2, Product4/2
  Abs/1 -> Scope1/1
  Gain3/1 -> Sum/1
  Gain6/1 -> Sum1/1
  Gain7/1 -> Sum2/1

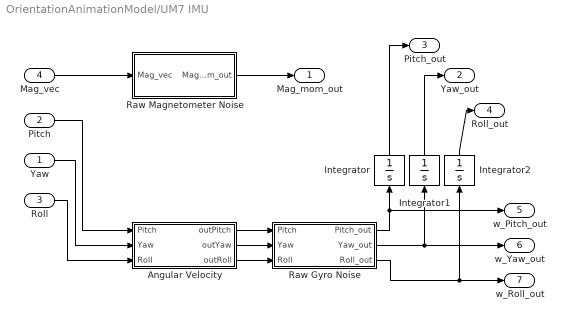
== system OrientationAnimationModel/UM7 IMU ==
  Yaw : Inport
  Pitch : Inport  Port=2
  Roll : Inport  Port=3
  Mag_vec : Inport  Port=4
  Angular Velocity : Subsystem  TreatAsAtomicUnit=on
  Integrator : Integrator
  Integrator1 : Integrator
  Integrator2 : Integrator
  Raw Gyro Noise : Subsystem  TreatAsAtomicUnit=on
  Raw Magnetometer Noise : Subsystem  TreatAsAtomicUnit=on
  Mag_mom_out : Outport
  Yaw_out : Outport  Port=2
  Pitch_out : Outport  Port=3
  Roll_out : Outport  Port=4
  w_Pitch_out : Outport  Port=5
  w_Yaw_out : Outport  Port=6
  w_Roll_out : Outport  Port=7
  wires:
  Pitch/1 -> Angular Velocity/1(Pitch)
  Yaw/1 -> Angular Velocity/2(Yaw)
  Roll/1 -> Angular Velocity/3(Roll)
  Mag_vec/1 -> Raw Magnetometer Noise/1(Mag_vec)
  Angular Velocity/1(outPitch) -> Raw Gyro Noise/1(Pitch)
  Angular Velocity/2(outYaw) -> Raw Gyro Noise/2(Yaw)
  Angular Velocity/3(outRoll) -> Raw Gyro Noise/3(Roll)
  Raw Magnetometer Noise/1(Mag_mom_out) -> Mag_mom_out/1
  Raw Gyro Noise/2(Yaw_out) -> w_Yaw_out/1, Integrator1/1
  Raw Gyro Noise/1(Pitch_out) -> w_Pitch_out/1, Integrator/1
  Raw Gyro Noise/3(Roll_out) -> w_Roll_out/1, Integrator2/1
  Integrator/1 -> Pitch_out/1
  Integrator1/1 -> Yaw_out/1
  Integrator2/1 -> Roll_out/1

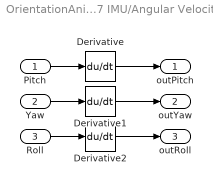
== system OrientationAnimationModel/UM7 IMU/Angular Velocity ==
  Pitch : Inport
  Yaw : Inport  Port=2
  Roll : Inport  Port=3
  Derivative : Derivative
  Derivative1 : Derivative
  Derivative2 : Derivative
  outPitch : Outport
  outYaw : Outport  Port=2
  outRoll : Outport  Port=3
  wires:
  Roll/1 -> Derivative2/1
  Yaw/1 -> Derivative1/1
  Pitch/1 -> Derivative/1
  Derivative/1 -> outPitch/1
  Derivative1/1 -> outYaw/1
  Derivative2/1 -> outRoll/1

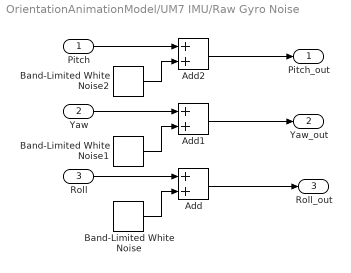
== system OrientationAnimationModel/UM7 IMU/Raw Gyro Noise ==
  Pitch : Inport
  Yaw : Inport  Port=2
  Roll : Inport  Port=3
  Add : Sum
  Add1 : Sum
  Add2 : Sum
  Band-Limited White Noise : simulink/Sources/Band-Limited White Noise  Cov=[0.0005]  Ts=0.1  seed=[23341]
  Band-Limited White Noise1 : simulink/Sources/Band-Limited White Noise  Cov=[0.0005]  Ts=0.1  seed=[23341]
  Band-Limited White Noise2 : simulink/Sources/Band-Limited White Noise  Cov=[0.0005]  Ts=0.1  seed=[23341]
  Pitch_out : Outport
  Yaw_out : Outport  Port=2
  Roll_out : Outport  Port=3
  wires:
  Band-Limited White Noise/1 -> Add/2
  Roll/1 -> Add/1
  Add/1 -> Roll_out/1
  Add1/1 -> Yaw_out/1
  Band-Limited White Noise1/1 -> Add1/2
  Yaw/1 -> Add1/1
  Add2/1 -> Pitch_out/1
  Band-Limited White Noise2/1 -> Add2/2
  Pitch/1 -> Add2/1

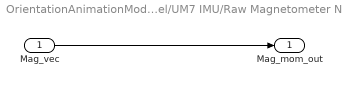
== system OrientationAnimationModel/UM7 IMU/Raw Magnetometer Noise ==
  Mag_vec : Inport
  Mag_mom_out : Outport
  wires:
  Mag_vec/1 -> Mag_mom_out/1

== matlab function OrientationAnimationModel/MATLAB Function ==
  data: Gamma output
function Gamma = fcn()

Gamma = [[0.04+6.25E-5,         0,                  0,                  6.25E-5,            0,              0       ];
         [0,                    0.05+6.25E-5,       0.02,               0,                  6.25E-5,        0       ];
         [0,                    0.02,               0.05+6.25E-5,       0,                  0,              6.25E-5 ];
         [6.25E-5,              0,                  0,                  6.25E-5,            0,              0       ];
         [0,                    6.25E-5,            0,                  0,                  6.25E-5,        0       ];
         [0,                    0,                  6.25E-5             0,                  0,              6.25E-5 ]];

== matlab function OrientationAnimationModel/MATLAB Function1 ==
  data: s input; y output; t input; I input; I_w input
function y = fcn(s, t, I, I_w)

w = [s(1); s(2); s(3)];
a1 = [1; 0; 0];
a2 = [0; 1; 0];
a3 = [0; 0; 1];
J = 6.25E-5;
part1 = -cross(w, I*w + a1*J*s(4) + a2*J*s(5) + a3*J*s(6) + I_w*w);
y = [part1(1); part1(2); part1(3); t(1); t(2); t(3)];

== matlab function OrientationAnimationModel/Subsystem3/Quat2Eigenaxis Rotation ==
  data: quat input; phi output; e output
function [phi, e] = fcn(quat)

e = [0;0;0];
phi = 0;

coder.extrinsic("quat2axang");
axang = quat2axang(reshape(quat,[1,4]));
%e = [axang(1,1), axang(1,2), axang(1,3)];
e = reshape([axang(1,1), axang(1,2), axang(1,3)],[3,1]);
phi = axang(1,4);


%e = reshape(e,[3,1]);

%e = [axang(0,1); axang(0,2); axang(0,3)];
%phi = axang(0,4);

== matlab function OrientationAnimationModel/Quaternion Calculations/Quaternion Derivative Matrix ==
  data: omega input; Omega output
function Omega = fcn(omega)

omega_cell = num2cell(omega);
[omega_x, omega_y, omega_z] = omega_cell{:};

%omega_x = omega(1);
%omega_y = omega(2);
%omega_z = omega(3);

Omega = [[0,            -omega_x,   -omega_y,   -omega_z];
         [omega_x,      0,          -omega_z,    omega_y];
         [omega_y,      omega_z,    0,          -omega_x];
         [omega_z,      -omega_y,   omega_x,    0       ]];

== matlab function OrientationAnimationModel/Subsystem4/MATLAB Function ==
  data: u input; y output
function y = fcn(u)

y = wrapToPi(u);
if y > pi/2
    y = pi - y;
end

== matlab function OrientationAnimationModel/Subsystem4/Quat2Eigenaxis Rotation ==
  data: quat input; phi output; e output
function [phi, e] = fcn(quat)

e = [0;0;0];
phi = 0;

coder.extrinsic("quat2axang");
axang = quat2axang(reshape(quat,[1,4]));
%e = [axang(1,1), axang(1,2), axang(1,3)];
e = reshape([axang(1,1), axang(1,2), axang(1,3)],[3,1]);
phi = axang(1,4);


%e = reshape(e,[3,1]);

%e = [axang(0,1); axang(0,2); axang(0,3)];
%phi = axang(0,4);
